simulink model "Arizona_base_GOAT_TjeerdRC"  (R2022a)
settings: Solver=FixedStepDiscrete  StartTime=0.0  StopTime=inf  FixedStep=Ts  RelTol=1e-3  EnableMultiTasking=on
undefined symbols (not defined in the file): DiscIntNeverNeededParam, Ended, IO307, N_Init, Nref, phd, phi_Init, Single, x_Init, y_Init
libraries: speedgoatlib_fpga_dio x30, speedgoatlib_fpga_quadrature x19, simulink x10, speedgoatlib_IO141 x9, xpcobsoletelib x7, cstblocks x5, speedgoatlib_fpga x3
(part 2 of 3)

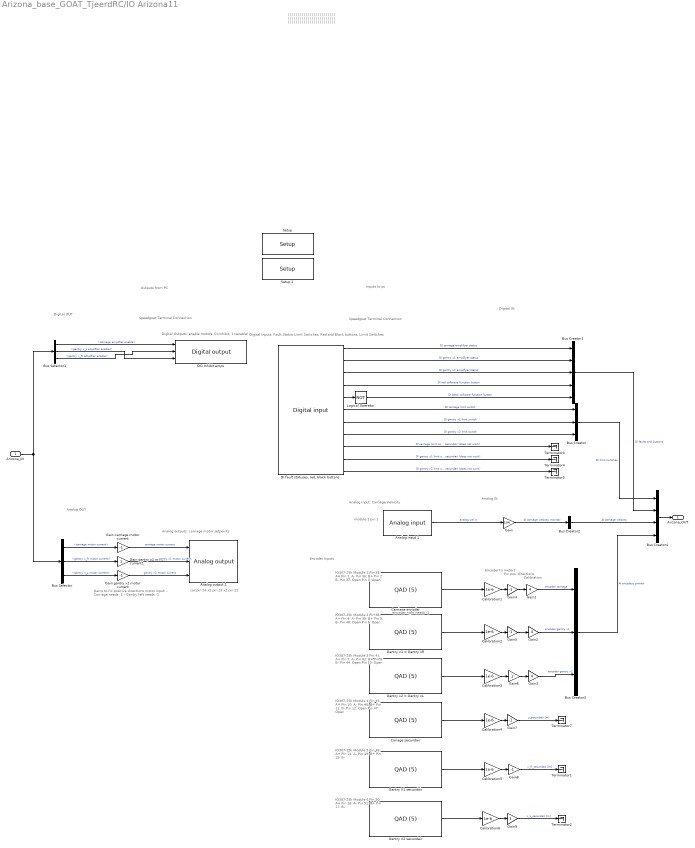
== system Arizona_base_GOAT_TjeerdRC/IO Arizona11 ==
  note: Fix pos.
      | directions
  note: Gains to fix positive directions motor input:
      | - Carriage needs -1
      | - Gantry left needs -1
  note: Inputs to pc
  note: Analog IN
  note: Digital IN
  note: Speedgoat Terminal Connection
  note: Outputs from PC
  note: Speedgoat Terminal Connection
  note: Digital Inputs: Fault Status Limit Switches, Red and Black buttons, Limit Switches
  note: Analog input: Carriage Velocity
  note: module 1
      | pin 1
  note: Digital OUT
  note: Analog OUT
  note: Analog outputs: carriage motor setpoints
  note: car pin 24
      | x1 pin 23
      | x2 pin 22
  note: |
      | |
      | |
      | |
      | |
      | |
      | |
      | |
      | |
      | |
      | |
      | |
      | |
      | |
      | |
      | |
      | |
      | |
      | |
      | |
      | |
      | |
      | |
      | |
      | |
      | |
      | |
      | |
      | |
      | |
      | |
      | |
      | |
      | |
      | |
      | |
      | |
      | |
      | |
      | |
      | |
      | |
      | |
      | |
      | |
      | |
      | |
      | |
      | |
      | |
      | |
      | |
      | |
      | |
      | |
      | |
      | |
      | |
      | |
      | |
      | |
      | |
      | |
      | |
      | |
      | |
      | |
      | |
      | |
      | |
      | |
      | |
  note: Digital Outputs: enable motors: 0=inhibit; 1=enable!
  note: Encoder
      | to meters
  note: Encoder Inputs
  note: encoder right needs -1
  note: IO307-25k
      | Module 4
      | Pin 45: A+
      | Pin 10: A-
      | Pin 46: B+
      | Pin 11: B-
      | Pin 12: Open
      | Pin 47: Open
  note: IO307-25k
      | Module 6
      | Pin 50: A+
      | Pin 16: A-
      | Pin 51: B+
      | Pin 17: B-
  note: IO307-25k
      | Module 3
      | Pin 41: A+
      | Pin 7: A-
      | Pin 42: B+
      | Pin 8: B-
      | Pin 44: Open
      | Pin 10: Open
  note: IO307-25k
      | Module 2
      | Pin 38: A+
      | Pin 4: A-
      | Pin 39: B+
      | Pin 5: B-
      | Pin 40: Open
      | Pin 6: Open
  note: IO307-25k
      | Module 5
      | Pin 48: A+
      | Pin 14: A-
      | Pin 49: B+
      | Pin 15: B-
  note: IO307-25k
      | Module 1
      | Pin 35: A+
      | Pin 1: A-
      | Pin 36: B+
      | Pin 2: B-
      | Pin 37: Open
      | Pin 3: Open
  note: Calibration
  Arizona_IN : Inport
  Analog input 1 : speedgoatlib_IO141/Analog input   parModuleId=1  parSampleTime=Ts  parPciSlot=-1  parAdcChannels=4  parAdcNumActiveChannels=[1 0]  parAdcVoltageRange=[5 5 5 5 5 5 5 5 5 5 5 5 5 5 5 5]  parAdcCoupling=[2 1]  parAdcContSampling=0  parAdcDmaEnable=0  parAdcActiveDmaDevices=[1 1 1 1]  parAdcFrameSize=100
      settings: SourceProductName=Simulink Real-Time: Speedgoat I/O Blockset
  Analog output 2 : speedgoatlib_IO141/Analog output   parModuleId=1  parSampleTime=Ts  parPciSlot=-1  parDacChannels=[1 2 3]  parDacVoltageRange=[5 5 5 7]  parDacOverRange=[0 0 0 0]  parDacInitValues=[0 0 0]  parDacReset=[1 1 1]  parDacSyncOut=1  parDacDmaEnable=0  parDacActiveDmaDevices=[1 1 1 1]  parDacDmaLatency=1  parDacFrameSize=100
      settings: SourceProductName=Simulink Real-Time: Speedgoat I/O Blockset
  Bus Creator : BusCreator  Inputs=3
  Bus Creator1 : BusCreator  Inputs=5
  Bus Creator2 : BusCreator  Inputs=1
  Bus Creator3 : BusCreator  Inputs=3
  Bus Creator4 : BusCreator  Inputs=4
  Bus Selector : BusSelector  OutputSignals=carriage motor current,gantry x_R motor current,gantry x_L motor current
  Bus Selector1 : BusSelector  OutputSignals=carriage amplifier enable,gantry x_L amplifier enable,gantry x_R amplifier enable
  Calibration{1..6} (6 alike) : Gain  Gain=1e-6
  Cariage secundair : speedgoatlib_fpga_quadrature/QAD (5)  id=1  chan=[4]  sampleTime=0.001  enableDma=on  board=Please select...  pciSlot=-1  numOfSlots=[1]  sensorType=Capture A + B Signal  interpolatePosition=off  swapAB=off  indexControlMode=Ignore Index  latchMode=Disabled  gateIndex=No Gating  speedFilterWidth=4  showInputSpeedFilterWidth=off  glitchFilterSeconds=106.7e-9  glitchFilterSecondsEff=108.5e-9  showInputClearPosition=off  showInputClearIndexFound=off  showOutputPosition=off  showOutputTurn=on  showOutputSpeed=off  showOutputIndexFound=off  showOutputLastPulse=off
      settings: SourceProductName=Simulink Real-Time: Speedgoat I/O Blockset
  Carriage encoder : speedgoatlib_fpga_quadrature/QAD (5)  id=1  chan=[1]  sampleTime=0.001  enableDma=on  board=Please select...  pciSlot=-1  numOfSlots=[1]  sensorType=Capture A + B Signal  interpolatePosition=off  swapAB=off  indexControlMode=Ignore Index  latchMode=Disabled  gateIndex=No Gating  speedFilterWidth=4  showInputSpeedFilterWidth=off  glitchFilterSeconds=106.7e-9  glitchFilterSecondsEff=108.5e-9  showInputClearPosition=off  showInputClearIndexFound=off  showOutputPosition=off  showOutputTurn=on  showOutputSpeed=off  showOutputIndexFound=off  showOutputLastPulse=off
      settings: SourceProductName=Simulink Real-Time: Speedgoat I/O Blockset
  "DI fault statuses, red, black buttons" : speedgoatlib_fpga_dio/Digital input  id=1  chan=[33:37,41:46]  ts=Ts  pciSlot=-1  board=IO307-25k  vectorizeOutput=off
      settings: SourceProductName=Simulink Real-Time: Speedgoat I/O Blockset
  DO Inhibit amps : speedgoatlib_fpga_dio/Digital output  id=1  chan=[30,31,32]  init=[0]  reset=[0]  vectorizeInput=off  ts=Ts  pciSlot=-1  board=Please select...
      settings: SourceProductName=Simulink Real-Time: Speedgoat I/O Blockset
  Gain : Gain  Gain=134
  Gain carriage motor current : Gain  Gain=-1
  Gain gantry x2 motor current : Gain  Gain=-1
  Gain gantry x2 motor current1 : Gain
  Gain1 : Gain  Gain=4
  Gain2 : Gain  Gain=4
  Gain3 : Gain  Gain=4
  Gain{4..5,7..8} (4 alike) : Gain  Gain=-1
  Gain6 : Gain
  Gain9 : Gain
  Gantry X1 secundair : speedgoatlib_fpga_quadrature/QAD (5)  id=1  chan=[5]  sampleTime=0.001  enableDma=on  board=Please select...  pciSlot=-1  numOfSlots=[1]  sensorType=Capture A + B Signal  interpolatePosition=off  swapAB=off  indexControlMode=Ignore Index  latchMode=Disabled  gateIndex=No Gating  speedFilterWidth=4  showInputSpeedFilterWidth=off  glitchFilterSeconds=106.7e-9  glitchFilterSecondsEff=108.5e-9  showInputClearPosition=off  showInputClearIndexFound=off  showOutputPosition=off  showOutputTurn=on  showOutputSpeed=off  showOutputIndexFound=off  showOutputLastPulse=off
      settings: SourceProductName=Simulink Real-Time: Speedgoat I/O Blockset
  Gantry x1 = Gantry xR : speedgoatlib_fpga_quadrature/QAD (5)  id=1  chan=[2]  sampleTime=0.001  enableDma=on  board=Please select...  pciSlot=-1  numOfSlots=[1]  sensorType=Capture A + B Signal  interpolatePosition=off  swapAB=off  indexControlMode=Ignore Index  latchMode=Disabled  gateIndex=No Gating  speedFilterWidth=4  showInputSpeedFilterWidth=off  glitchFilterSeconds=106.7e-9  glitchFilterSecondsEff=108.5e-9  showInputClearPosition=off  showInputClearIndexFound=off  showOutputPosition=off  showOutputTurn=on  showOutputSpeed=off  showOutputIndexFound=off  showOutputLastPulse=off
      settings: SourceProductName=Simulink Real-Time: Speedgoat I/O Blockset
  Gantry x2 = Gantry xL : speedgoatlib_fpga_quadrature/QAD (5)  id=1  chan=[3]  sampleTime=0.001  enableDma=on  board=Please select...  pciSlot=-1  numOfSlots=[1]  sensorType=Capture A + B Signal  interpolatePosition=off  swapAB=off  indexControlMode=Ignore Index  latchMode=Disabled  gateIndex=No Gating  speedFilterWidth=4  showInputSpeedFilterWidth=off  glitchFilterSeconds=106.7e-9  glitchFilterSecondsEff=108.5e-9  showInputClearPosition=off  showInputClearIndexFound=off  showOutputPosition=off  showOutputTurn=on  showOutputSpeed=off  showOutputIndexFound=off  showOutputLastPulse=off
      settings: SourceProductName=Simulink Real-Time: Speedgoat I/O Blockset
  Gentry X2 secundair : speedgoatlib_fpga_quadrature/QAD (5)  id=1  chan=[6]  sampleTime=0.001  enableDma=on  board=Please select...  pciSlot=-1  numOfSlots=[1]  sensorType=Capture A + B Signal  interpolatePosition=off  swapAB=off  indexControlMode=Ignore Index  latchMode=Disabled  gateIndex=No Gating  speedFilterWidth=4  showInputSpeedFilterWidth=off  glitchFilterSeconds=106.7e-9  glitchFilterSecondsEff=108.5e-9  showInputClearPosition=off  showInputClearIndexFound=off  showOutputPosition=off  showOutputTurn=on  showOutputSpeed=off  showOutputIndexFound=off  showOutputLastPulse=off
      settings: SourceProductName=Simulink Real-Time: Speedgoat I/O Blockset
  Logical Operator : Logic  Operator=NOT  AllPortsSameDT=off  OutDataTypeStr=boolean
  Setup : speedgoatlib_fpga/Setup/Setup  board=IO307-25k  id=1  device_id=1  frontIO=None  rearIO=None  bitstreamFile=speedgoat_IO307_25k_CI_02479  rev=1.000000  timestamp_string=28/12/21 17:14:03  fpgaFreq=73.73 MHz  fpgaTick=13.56 ns  ProgSpiFlash=off  ProgBPIFlash=off  pciSlot=-1  PullRPort0=pull-up 3.3V  VioPort0=3.3V  PullRPort1=pull-up 3.3V  VioPort1=3.3V  PullRPort2=pull-up 3.3V  VioPort2=3.3V  PullRPort3=pull-up 3.3V  VioPort3=3.3V  PullRPort4=pull-up 3.3V  VioPort4=3.3V  PullRPort5=pull-up 3.3V  VioPort5=3.3V  PullRPort6=pull-up 3.3V  VioPort6=3.3V  PullRPort15=pull-up 3.3V  PullRPort31=pull-up 3.3V  PullRPort47=pull-up 3.3V  PullRPort63=pull-up 3.3V  diffLineTermination_1=on  diffLineTermination_2=on  diffLineTermination_3=on  diffLineTermination_4=on  diffLineTermination_5=on  diffLineTermination_6=on  diffLineTermination_7=on  diffLineTermination_8=on
      settings: SourceProductName=Simulink Real-Time: Speedgoat I/O Blockset
  Setup 2 : speedgoatlib_IO141/Setup   parPciSlot=-1  parModuleId=1  parInterModuleSync=Independent  parConvClockBaseRate=20MHz  parConvClock1Divider=20000  parConvClock2Divider=20000  parFrameTriggerEnable=off  parFrameTriggerDivider=10  parConvClock1BaseRate=1  parConvClock2BaseRate=1  parFrameTriggerClock=1  parAdcCoupling1=Single-Ended  parAdcChannels1=[1 2]  parAdcChannel11=off  parAdcChannel12=off  parAdcChannel13=off  parAdcChannel14=on  parAdcChannel15=off  parAdcChannel16=off  parAdcChannel17=off  parAdcChannel18=off  parAdcRangeAll1=+-10.24 V  parVoltageRangePerChannelEn1=off  parAdcRange11=+-0.64 V  parAdcRange12=+-0.64 V  parAdcRange13=+-0.64 V  parAdcRange14=+-0.64 V  parAdcRange15=+-0.64 V  parAdcRange16=+-0.64 V  parAdcRange17=+-0.64 V  parAdcRange18=+-0.64 V  parAdcCoupling2=Differential  parAdcChannels2=[9 10]  parAdcChannel21=off  parAdcChannel22=off  parAdcChannel23=off  parAdcChannel24=off  parAdcChannel25=off  parAdcChannel26=off  parAdcChannel27=off  parAdcChannel28=off  parAdcRangeAll2=+-10.24 V  parVoltageRangePerChannelEn2=off  parAdcRange21=+-0.64 V  parAdcRange22=+-0.64 V  parAdcRange23=+-0.64 V  parAdcRange24=+-0.64 V  parAdcRange25=+-0.64 V  parAdcRange26=+-0.64 V  parAdcRange27=+-0.64 V  parAdcRange28=+-0.64 V  parAdcChannels=4  parAdcNumActiveChannels=[1 0]  parAdcVoltageRange=[5 5 5 5 5 5 5 5 5 5 5 5 5 5 5 5]  parAdcCoupling=[2 1]  parAdcContSampling=off  parAdcAutoCorrection=on  parAdcDmaEnable=off  parAdcDmaClock=Clock 1  parAdcFrameSize_=100  parAdcSampleTime_=-1  parAdcActiveDmaDevices=[1 1 1 1]  parAdcFrameTriggerEnable=0  parAdcFrameSize=100  parAdcSampleTime=0.1  parDacChannels=[1 2]  parDacChannel1=on  parDacChannel2=on  parDacChannel3=on  parDacChannel4=off  parDacInitValues=0  parDacResets=1  parDacVoltageRange=[5 5 5 7]  parDacOverRange=[0 0 0 0]  parDacRange1=+-5 V  parDacInitValue1=0  parDacReset1=on  parDacRange2=+-5 V  parDacInitValue2=0  parDacReset2=on  parDacRange3=+-5 V  parDacInitValue3=0  parDacReset3=on  parDacRange4=+-10 V  parDacInitValue4=0  parDacReset4=on  parDacAutoCorrection=on  parDacSyncOut=on  parDacDmaEnable=off  parDacDmaLatency=As small as possible  parDacDmaClock=Clock 1  parDacFrameSize_=100  parDacSampleTime_=-1  parDacActiveDmaDevices=[1 1 1 1]  parDacFrameTriggerEnable=0  parDacFrameSize=100  parDacSampleTime=0.1  parDiChannels=[1 2 3 4 5]  parDoChannels=[6 7 8]  parDioChannel1=In  parDioChannel2=In  parDioChannel3=In  parDioChannel4=In  parDioChannel5=In  parDioChannel6=Out  parDioChannel7=Out  parDioChannel8=Out  parDoInitValues=[0 0 0]  parDoReset=[1 1 1]  parDoInitValue1=0  parDoReset1=on  parDoInitValue2=0  parDoReset2=on  parDoInitValue3=0  parDoReset3=on  parDoInitValue4=0  parDoReset4=on  parDoInitValue5=0  parDoReset5=on  parDoInitValue6=0  parDoReset6=on  parDoInitValue7=0  parDoReset7=on  parDoInitValue8=0  parDoReset8=on  parDiDebounceEnable=off  parDiDebounceTime=0  parDiDebounceValue=0  parDioPullRefFront=Pull-up 3.3 V  parDioPullRefRear=Floating
      settings: SourceProductName=Simulink Real-Time: Speedgoat I/O Blockset
  Terminator{1..5,7} (6 alike) : Terminator
  Arizona_OUT : Outport
  wires:
  "DI fault statuses, red, black buttons"/8 -> Bus Creator/3  "DI gantry x2 limit switch"
  Bus Creator3/1 -> Bus Creator4/4  "AI encoders primair"
  Bus Creator2/1 -> Bus Creator4/3  "AI carriage velocity"
  Bus Creator1/1 -> Bus Creator4/2  "DI faults and buttons"
  Bus Creator/1 -> Bus Creator4/1  "DI limit switches"
  Gain carriage motor current/1 -> Analog output 2/1  "carriage motor current"
  Bus Selector/3 -> Gain gantry x2 motor current/1  "<gantry x_L motor current>"
  "DI fault statuses, red, black buttons"/5 -> Logical Operator/1
  Logical Operator/1 -> Bus Creator1/5  "DI black sofware function button"
  "DI fault statuses, red, black buttons"/2 -> Bus Creator1/2  "DI gantry x1 amplifyer status"
  "DI fault statuses, red, black buttons"/3 -> Bus Creator1/3  "DI gantry x2 amplifyer status"
  Bus Selector/2 -> Gain gantry x2 motor current1/1  "<gantry x_R motor current>"
  "DI fault statuses, red, black buttons"/4 -> Bus Creator1/4  "DI red software function button"
  "DI fault statuses, red, black buttons"/7 -> Bus Creator/2  "DI gantry x1 limit switch"
  "DI fault statuses, red, black buttons"/1 -> Bus Creator1/1  "DI carriage amplifyer status"
  "DI fault statuses, red, black buttons"/6 -> Bus Creator/1  "DI carriage limit switch"
  Bus Selector/1 -> Gain carriage motor current/1  "<carriage motor current>"
  Gain gantry x2 motor current/1 -> Analog output 2/3  "gantry x2 motor current"
  Gain/1 -> Bus Creator2/1  "AI carriage velocity monitor"
  Bus Creator4/1 -> Arizona_OUT/1
  Gain gantry x2 motor current1/1 -> Analog output 2/2  "gantry x1 motor current"
  Analog input 1/1 -> Gain/1  "analog vel in"
  Bus Selector1/3 -> DO Inhibit amps/2  "<gantry x_R amplifier enable>"
  Arizona_IN/1 -> Bus Selector1/1, Bus Selector/1
  Bus Selector1/1 -> DO Inhibit amps/1  "<carriage amplifier enable>"
  Calibration2/1 -> Gain5/1
  Calibration3/1 -> Gain6/1
  Calibration1/1 -> Gain4/1
  Calibration4/1 -> Gain7/1
  Calibration5/1 -> Gain8/1
  Calibration6/1 -> Gain9/1
  "DI fault statuses, red, black buttons"/9 -> Terminator3/1  "DI carriage limit switch secundair (does not work)"
  "DI fault statuses, red, black buttons"/10 -> Terminator4/1  "DI gantry x1 limit switch secundair (does not work)"
  "DI fault statuses, red, black buttons"/11 -> Terminator5/1  "DI gantry x2 limit switch secundair (does not work)"
  Bus Selector1/2 -> DO Inhibit amps/3  "<gantry x_L amplifier enable>"
  Gain2/1 -> Bus Creator3/2  "encoder gantry x1"
  Gain3/1 -> Bus Creator3/3  "encoder gantry x2"
  Gain8/1 -> Terminator1/1  "x_R_secundair [m]"
  Gain9/1 -> Terminator2/1  "x_L_secundair [m]"
  Gain1/1 -> Bus Creator3/1  "encoder carriage"
  Gain7/1 -> Terminator7/1  "y_secundair [m]"
  Carriage encoder/1 -> Calibration1/1
  Gantry x1 = Gantry xR/1 -> Calibration2/1
  Gantry x2 = Gantry xL/1 -> Calibration3/1
  Cariage secundair/1 -> Calibration4/1
  Gantry X1 secundair/1 -> Calibration5/1
  Gentry X2 secundair/1 -> Calibration6/1
  Gain4/1 -> Gain1/1
  Gain5/1 -> Gain2/1
  Gain6/1 -> Gain3/1

== system Arizona_base_GOAT_TjeerdRC/Penholder mechanism1 ==
  note: -1= naar beneden
      | 1= omhoog
      | 0=uit
  note: -1=CCW
      | 1= CW
      | 0=uit
  note: LimitSwitch_z_up DI PF50 PIN 6 #CON-0 6229
  note: Limitswitch_z_down DI PFI14 PIN 1 #CON-0 6229
  note: LimitSwitch_Theta DI PFI9 PIN 3 #CON-0 6229
  Change color : Inport
  homingDone : Inport  Port=2
  Change color Chart : Stateflow chart  TreatAsAtomicUnit=on
  Data Type Conversion1 : DataTypeConversion  SaturateOnIntegerOverflow=off  RndMeth=Floor
  Data Type Conversion2 : DataTypeConversion  SaturateOnIntegerOverflow=off  RndMeth=Floor
  Data Type Conversion3 : DataTypeConversion  SaturateOnIntegerOverflow=off  RndMeth=Floor
  Gain on phi2 : Gain  Gain=0.07
  Gain on phi3 : Gain
  Motor Theta : Subsystem
  Motor Z : Subsystem
  "PCI 6229 PFI DI " : xpcobsoletelib/Obsolete  Commented=on
      settings: SourceProductBaseCode=XP
  PCI 6229 PFI DI 1 : xpcobsoletelib/Obsolete  Commented=on
      settings: SourceProductBaseCode=XP
  PCI 6229 PFI DI 2 : xpcobsoletelib/Obsolete  Commented=on
      settings: SourceProductBaseCode=XP
  log_jogspeed : Gain
  Penholder_active : Outport
  wires:
  ? -> Data Type Conversion1/1
  ? -> Data Type Conversion2/1
  Gain on phi2/1 -> Motor Theta/1(v_theta in mm/s)
  Gain on phi3/1 -> Motor Z/1(v_Z in mm/s)
  ? -> Data Type Conversion3/1
  Data Type Conversion3/1 -> Change color Chart/4(limitSwitch_Theta)
  Change color/1 -> Change color Chart/1(change_color)
  Change color Chart/1(jogspeed_Z) -> Gain on phi3/1
  Change color Chart/2(jogspeed_Theta) -> log_jogspeed/1
  Data Type Conversion2/1 -> Change color Chart/2(limitSwitch_z_up)
  Data Type Conversion1/1 -> Change color Chart/3(limitSwitch_z_down)
  Change color Chart/3(active) -> Penholder_active/1
  log_jogspeed/1 -> Gain on phi2/1  "jogSpeed"
  homingDone/1 -> Change color Chart/5(homingDone)

== system Arizona_base_GOAT_TjeerdRC/Repetitive Controller ==
  Learning Gain : Inport
  y : Inport  Port=2
  r : Inport  Port=3
  e : Inport  Port=4
  Enable : EnablePort
  Lc : cstblocks/LTI System  sys=Lc  IC=[]
  Product : Product
  Qc : cstblocks/LTI System  sys=Qc  IC=[]
  Sum : Sum  Inputs=|++
  z^(N-phd-p_Q) : Delay  DelayLength=Nlength-phd-p_Q
  z^-phd : Delay  DelayLength=phd
  Out1 : Outport
  wires:
  Sum/1 -> z^(N-phd-p_Q)/1
  e/1 -> Sum/1
  z^(N-phd-p_Q)/1 -> Qc/1
  Qc/1 -> z^-phd/1, Lc/1
  z^-phd/1 -> Sum/2
  Lc/1 -> Product/2
  Product/1 -> Out1/1
  Learning Gain/1 -> Product/1

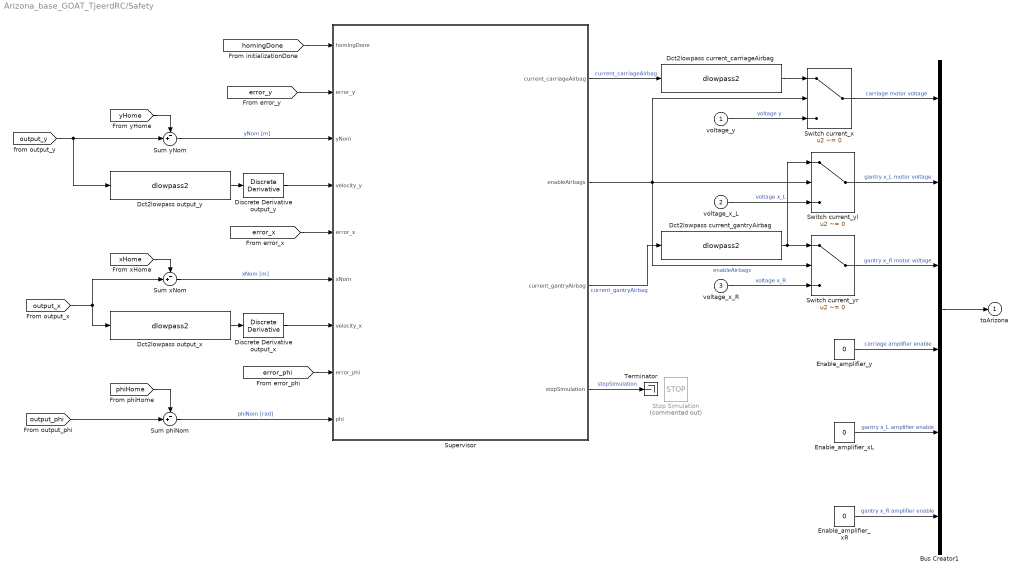
== system Arizona_base_GOAT_TjeerdRC/Safety ==
  voltage_y : Inport
  voltage_x_L : Inport  Port=2
  voltage_x_R : Inport  Port=3
  Bus Creator1 : BusCreator  Inputs=carriage motor voltage,gantry x_L motor voltage,gantry x_R motor voltage,carriage amplifier enable,gantry x_L amplifier enable,gantry x_R amplifier enable
  Dct2lowpass current_carriageAirbag : S-Function  FunctionName=dlowpass2  Parameters=f_den, b_den, 0.001  SFunctionDeploymentMode=off  EnableBusSupport=off  mask(dctools){f_den=5, b_den=2}
      mask prompts: f_den "Pole [Hz]"; b_den "Damping pole [-]"
      mask help: This block implements a discrete time 2nd order lowpass filter.
      mask Display: disp('DCT 2nd order lowpass')
  Dct2lowpass current_gantryAirbag : S-Function  FunctionName=dlowpass2  Parameters=f_den, b_den, 0.001  SFunctionDeploymentMode=off  EnableBusSupport=off  mask(dctools){f_den=5, b_den=2}
      mask prompts: f_den "Pole [Hz]"; b_den "Damping pole [-]"
      mask help: This block implements a discrete time 2nd order lowpass filter.
      mask Display: disp('DCT 2nd order lowpass')
  Dct2lowpass output_x : S-Function  FunctionName=dlowpass2  Parameters=f_den, b_den, 0.001  SFunctionDeploymentMode=off  EnableBusSupport=off  mask(dctools){f_den=10, b_den=2}
      mask prompts: f_den "Pole [Hz]"; b_den "Damping pole [-]"
      mask help: This block implements a discrete time 2nd order lowpass filter.
      mask Display: disp('DCT 2nd order lowpass')
  Dct2lowpass output_y : S-Function  FunctionName=dlowpass2  Parameters=f_den, b_den, 0.001  SFunctionDeploymentMode=off  EnableBusSupport=off  mask(dctools){f_den=10, b_den=2}
      mask prompts: f_den "Pole [Hz]"; b_den "Damping pole [-]"
      mask help: This block implements a discrete time 2nd order lowpass filter.
      mask Display: disp('DCT 2nd order lowpass')
  Discrete Derivative output_x : simulink/Discrete/Discrete Derivative  gainval=1.0  ICPrevScaledInput=0.0  OutMin=[]  OutMax=[]  OutDataType=fixdt(1, 16)  OutScaling=2^-10  DoSatur=off
  Discrete Derivative output_y : simulink/Discrete/Discrete Derivative  gainval=1.0  ICPrevScaledInput=0.0  OutMin=[]  OutMax=[]  OutDataType=fixdt(1, 16)  OutScaling=2^-10  DoSatur=off
  Enable_amplifier_xL : Constant  Value=0
  Enable_amplifier_xR : Constant  Value=0
  Enable_amplifier_y : Constant  Value=0
  Stop Simulation : Stop  Commented=on
  Sum phiNom : Sum  Inputs=-+|
  Sum xNom : Sum  Inputs=-+|
  Sum yNom : Sum  Inputs=-+|
  Supervisor : Stateflow chart  TreatAsAtomicUnit=on
  Switch current_x : Switch  Criteria=u2 ~= 0  SaturateOnIntegerOverflow=off  InputSameDT=off
  Switch current_yl : Switch  Criteria=u2 ~= 0  SaturateOnIntegerOverflow=off  InputSameDT=off
  Switch current_yr : Switch  Criteria=u2 ~= 0  SaturateOnIntegerOverflow=off  InputSameDT=off
  Terminator : Terminator
  toArizona : Outport
  wires:
  [phiHome] -> Sum phiNom/1
  Sum phiNom/1 -> Supervisor/9(phi)  "phiNom [rad]"
  voltage_x_L/1 -> Switch current_yl/3  "voltage x_L"
  voltage_x_R/1 -> Switch current_yr/3  "voltage x_R"
  Dct2lowpass current_carriageAirbag/1 -> Switch current_x/1
  Dct2lowpass current_gantryAirbag/1 -> Switch current_yl/1, Switch current_yr/1
  Supervisor/3(current_gantryAirbag) -> Dct2lowpass current_gantryAirbag/1  "current_gantryAirbag"
  Discrete Derivative output_x/1 -> Supervisor/7(velocity_x)
  [xHome] -> Sum xNom/1
  Dct2lowpass output_x/1 -> Discrete Derivative output_x/1
  Sum xNom/1 -> Supervisor/6(xNom)  "xNom [m]"
  [output_x] -> Sum xNom/2, Dct2lowpass output_x/1
  [error_phi] -> Supervisor/8(error_phi)
  [error_x] -> Supervisor/5(error_x)
  Supervisor/2(enableAirbags) -> Switch current_yr/2, Switch current_yl/2, Switch current_x/2  "enableAirbags"
  Supervisor/1(current_carriageAirbag) -> Dct2lowpass current_carriageAirbag/1  "current_carriageAirbag"
  [error_y] -> Supervisor/2(error_y)
  Switch current_x/1 -> Bus Creator1/1  "carriage motor voltage"
  [homingDone] -> Supervisor/1(homingDone)
  [yHome] -> Sum yNom/1
  voltage_y/1 -> Switch current_x/3  "voltage y"
  Discrete Derivative output_y/1 -> Supervisor/4(velocity_y)
  Dct2lowpass output_y/1 -> Discrete Derivative output_y/1
  Sum yNom/1 -> Supervisor/3(yNom)  "yNom [m]"
  [output_y] -> Dct2lowpass output_y/1, Sum yNom/2
  Bus Creator1/1 -> toArizona/1
  Enable_amplifier_xL/1 -> Bus Creator1/5  "gantry x_L amplifier enable"
  Enable_amplifier_xR/1 -> Bus Creator1/6  "gantry x_R amplifier enable"
  Switch current_yl/1 -> Bus Creator1/2  "gantry x_L motor voltage"
  Enable_amplifier_y/1 -> Bus Creator1/4  "carriage amplifier enable"
  Switch current_yr/1 -> Bus Creator1/3  "gantry x_R motor voltage"
  [output_phi] -> Sum phiNom/2
  Supervisor/4(stopSimulation) -> Terminator/1  "stopSimulation"

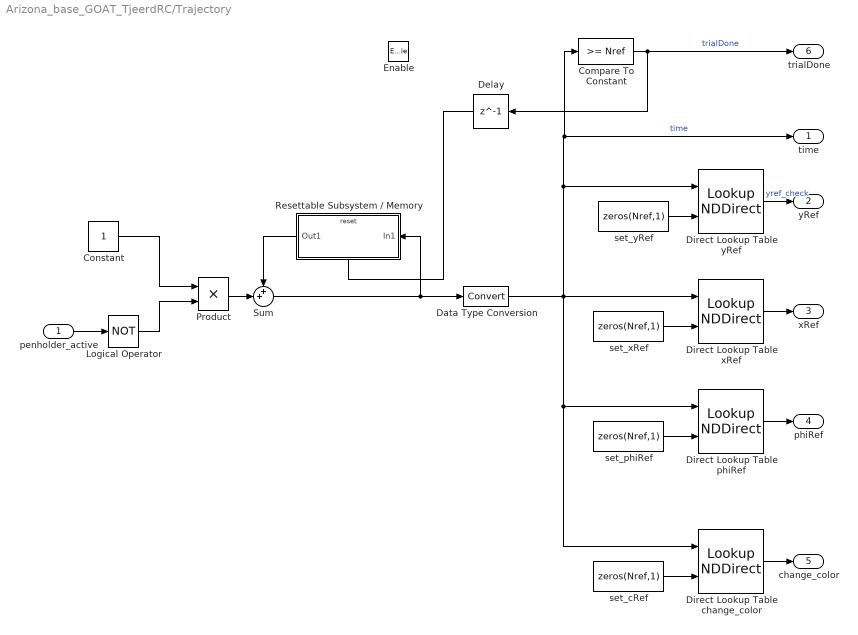
== system Arizona_base_GOAT_TjeerdRC/Trajectory ==
  penholder_active : Inport
  Enable : EnablePort  StatesWhenEnabling=reset
  Compare To Constant : simulink/Logic and Bit Operations/Compare To Constant  relop=>=  const=Nref  OutDataTypeStr=boolean
  Constant : Constant
  Data Type Conversion : DataTypeConversion  SaturateOnIntegerOverflow=off  RndMeth=Floor
  Delay : Delay  DelayLength=1  InitialCondition=0
  Direct Lookup Table change_color : LookupNDDirect  NumberOfTableDimensions=1  TableIsInput=on  Table=[4 5 ;16 19 ]
  Direct Lookup Table phiRef : LookupNDDirect  NumberOfTableDimensions=1  TableIsInput=on  Table=[4 5 ;16 19 ]
  Direct Lookup Table xRef : LookupNDDirect  NumberOfTableDimensions=1  TableIsInput=on  Table=[4 5 ;16 19 ]
  Direct Lookup Table yRef : LookupNDDirect  NumberOfTableDimensions=1  TableIsInput=on  Table=[4 5 ;16 19 ]
  Logical Operator : Logic  Operator=NOT  AllPortsSameDT=off  OutDataTypeStr=boolean
  Product : Product
  Resettable Subsystem / Memory : Subsystem  TreatAsAtomicUnit=on
  Sum : Sum  Inputs=++|
  set_cRef : Constant  Value=zeros(Nref,1)
  set_phiRef : Constant  Value=zeros(Nref,1)
  set_xRef : Constant  Value=zeros(Nref,1)
  set_yRef : Constant  Value=zeros(Nref,1)
  time : Outport
  yRef : Outport  Port=2
  xRef : Outport  Port=3
  phiRef : Outport  Port=4
  change_color : Outport  Port=5
  trialDone : Outport  Port=6
  wires:
  Direct Lookup Table phiRef/1 -> phiRef/1
  Direct Lookup Table yRef/1 -> yRef/1  "yref_check"
  Direct Lookup Table xRef/1 -> xRef/1
  set_yRef/1 -> Direct Lookup Table yRef/2
  set_xRef/1 -> Direct Lookup Table xRef/2
  Data Type Conversion/1 -> Compare To Constant/1, time/1, Direct Lookup Table yRef/1, Direct Lookup Table xRef/1, Direct Lookup Table change_color/1, Direct Lookup Table phiRef/1  "time"
  set_phiRef/1 -> Direct Lookup Table phiRef/2
  Constant/1 -> Product/1
  Sum/1 -> Resettable Subsystem / Memory/1(In1), Data Type Conversion/1
  penholder_active/1 -> Logical Operator/1
  Logical Operator/1 -> Product/2
  Direct Lookup Table change_color/1 -> change_color/1
  set_cRef/1 -> Direct Lookup Table change_color/2
  Compare To Constant/1 -> Delay/1, trialDone/1  "trialDone"
  Product/1 -> Sum/2
  Resettable Subsystem / Memory/1(Out1) -> Sum/1
  Delay/1 -> Resettable Subsystem / Memory/Reset

== system Arizona_base_GOAT_TjeerdRC/Homing/Enabled subsystem ==
  encoderSignals : Inport
  penholder_active : Inport  Port=2
  Enable : EnablePort  StatesWhenEnabling=reset
  Add phiHome : Sum  Inputs=|++
  Add xHome : Sum  Inputs=|++
  Add yHome : Sum  Inputs=|++
  Initialization : Subsystem
  Reset : Subsystem
  yHome : Outport
  xHome : Outport  Port=2
  phiHome : Outport  Port=3
  homingDone : Outport  Port=4  InitialOutput=0
  change_color : Outport  Port=5
  wires:
  encoderSignals/1 -> Reset/1(encoderSignals)
  Reset/1(yReset) -> Add yHome/1  "yReset"
  Reset/2(xReset) -> Add xHome/1  "xReset"
  Reset/3(phiReset) -> Add phiHome/1  "phiReset"
  Initialization/4(initializationDone) -> homingDone/1
  Add xHome/1 -> xHome/1
  Add yHome/1 -> yHome/1
  Add phiHome/1 -> phiHome/1
  penholder_active/1 -> Reset/2(penholder_active)
  Reset/5(change_color) -> change_color/1
  Initialization/3(phiInit) -> Add phiHome/2  "phiInit"
  Initialization/1(yInit) -> Add yHome/2  "yInit"
  Initialization/2(xInit) -> Add xHome/2  "xInit"
  Reset/4(resetDone) -> Initialization/1(resetDone)  "resetDone"

== system Arizona_base_GOAT_TjeerdRC/Homing/Memory block for homing during trials ==
  yHome : Inport
  xHome : Inport  Port=2
  phiHome : Inport  Port=3
  homeTrigger : Inport  Port=4
  Memory_phi : Subsystem
  Memory_x : Subsystem
  Memory_y : Subsystem
  yHome_memory : Outport
  xHome_memory : Outport  Port=2
  phiHome_memory : Outport  Port=3
  wires:
  yHome/1 -> Memory_y/2(yHome)
  xHome/1 -> Memory_x/2(xHome)
  phiHome/1 -> Memory_phi/2(phiHome)
  homeTrigger/1 -> Memory_phi/1(homeTrigger), Memory_x/1(homeTrigger), Memory_y/1(homeTrigger)
  Memory_y/1(Out1) -> yHome_memory/1
  Memory_x/1(1) -> xHome_memory/1
  Memory_phi/1(1) -> phiHome_memory/1

== system Arizona_base_GOAT_TjeerdRC/Homing old/Enabled subsystem ==
  encoderSignals : Inport
  penholder_active : Inport  Port=2
  Enable : EnablePort  StatesWhenEnabling=reset
  Add phiHome : Sum  Inputs=|++
  Add xHome : Sum  Inputs=|++
  Add yHome : Sum  Inputs=|++
  Initialization : Subsystem  TreatAsAtomicUnit=on
  Reset : Subsystem
  yHome : Outport
  xHome : Outport  Port=2
  phiHome : Outport  Port=3
  homingDone : Outport  Port=4  InitialOutput=0
  change_color : Outport  Port=5
  wires:
  encoderSignals/1 -> Reset/1(encoderSignals)
  Reset/4(resetDone) -> Initialization/Enable
  Reset/1(yReset) -> Add yHome/1  "yReset"
  Reset/2(xReset) -> Add xHome/1  "xReset"
  Reset/3(phiReset) -> Add phiHome/1  "phiReset"
  Initialization/4(initializationDone) -> homingDone/1
  Add xHome/1 -> xHome/1
  Add yHome/1 -> yHome/1
  Add phiHome/1 -> phiHome/1
  penholder_active/1 -> Reset/2(penholder_active)
  Reset/5(change_color) -> change_color/1
  Initialization/3(phiInit) -> Add phiHome/2  "phiInit"
  Initialization/1(yInit) -> Add yHome/2  "yInit"
  Initialization/2(xInit) -> Add xHome/2  "xInit"

== system Arizona_base_GOAT_TjeerdRC/Homing old/Memory ==
  homeTrigger : Inport
  yHome : Inport  Port=2
  Delay : Delay  DelayLength=1
  Memory : Memory
  Sum : Sum  Inputs=|++
  Switch : Switch  Criteria=u2 > Threshold  Threshold=1  SaturateOnIntegerOverflow=off  InputSameDT=off
  Switch1 : Switch  Criteria=u2 > Threshold  SaturateOnIntegerOverflow=off  InputSameDT=off
  Out1 : Outport
  wires:
  Switch/1 -> Memory/1
  Memory/1 -> Switch/3, Switch1/3, Sum/2
  homeTrigger/1 -> Delay/1, Switch1/2
  yHome/1 -> Sum/1
  Sum/1 -> Switch1/1
  Switch1/1 -> Switch/1, Out1/1
  Delay/1 -> Switch/2

== system Arizona_base_GOAT_TjeerdRC/Penholder mechanism1/Motor Theta ==
  note: enable DO PFI4 PIN 41 #CON-0 6229
  note: direction DO PFI3 PIN 42 #CON-0 6229
  v_theta in mm/s : Inport
  Abs : Abs  SaturateOnIntegerOverflow=off
  Compare To Zero : simulink/Logic and Bit Operations/Compare To Zero  relop=>  OutDataTypeStr=boolean
  Data Type Conversion : DataTypeConversion  SaturateOnIntegerOverflow=off  RndMeth=Floor
  "PCI 6229 PFI DO " : xpcobsoletelib/Obsolete  Commented=on
      settings: SourceProductBaseCode=XP
  PCI 6229 PWM Generate Chan 0 : xpcobsoletelib/Obsolete  Commented=on
      settings: SourceProductBaseCode=XP
  PWMcreator5 : Subsystem
  wires:
  PWMcreator5/1(HighSamples) -> ?
  PWMcreator5/2(LowSamples) -> ?
  Compare To Zero/1 -> Data Type Conversion/1
  PWMcreator5/3(DirectionBit) -> ?
  Data Type Conversion/1 -> ?
  Abs/1 -> Compare To Zero/1
  v_theta in mm/s/1 -> Abs/1, PWMcreator5/1(velocity [mm / s])

== system Arizona_base_GOAT_TjeerdRC/Penholder mechanism1/Motor Z ==
  note: enable DO PFI11 PIN 46 #CON-0 6229
  note: direction DO PFI10 PIN 45 #CON-0 6229
  v_Z in mm/s : Inport
  Abs1 : Abs  SaturateOnIntegerOverflow=off
  Compare To Zero1 : simulink/Logic and Bit Operations/Compare To Zero  relop=>  OutDataTypeStr=boolean
  Data Type Conversion1 : DataTypeConversion  SaturateOnIntegerOverflow=off  RndMeth=Floor
  PCI 6229 PFI DO 1 : xpcobsoletelib/Obsolete  Commented=on
      settings: SourceProductBaseCode=XP
  PCI 6229 PWM Generate Chan 1 : xpcobsoletelib/Obsolete  Commented=on
      settings: SourceProductBaseCode=XP
  PWMcreator1 : Subsystem
  wires:
  PWMcreator1/1(HighSamples) -> ?
  PWMcreator1/2(LowSamples) -> ?
  Compare To Zero1/1 -> Data Type Conversion1/1
  PWMcreator1/3(DirectionBit) -> ?
  v_Z in mm/s/1 -> Abs1/1, PWMcreator1/1(velocity [mm / s])
  Data Type Conversion1/1 -> ?
  Abs1/1 -> Compare To Zero1/1

== system Arizona_base_GOAT_TjeerdRC/Trajectory/Resettable Subsystem // Memory ==
  In1 : Inport
  Reset : ResetPort  DisableCoverage=on
  Memory : Memory
  Out1 : Outport
  wires:
  In1/1 -> Memory/1
  Memory/1 -> Out1/1

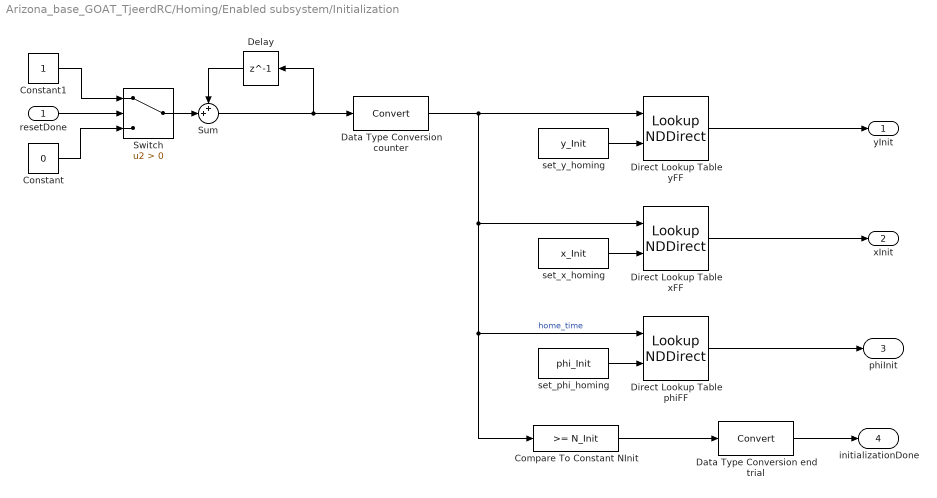
== system Arizona_base_GOAT_TjeerdRC/Homing/Enabled subsystem/Initialization ==
  resetDone : Inport
  Compare To Constant NInit : simulink/Logic and Bit Operations/Compare To Constant  relop=>=  const=N_Init  OutDataTypeStr=boolean
  Constant : Constant  Value=0
  Constant1 : Constant
  Data Type Conversion counter : DataTypeConversion  SaturateOnIntegerOverflow=off  RndMeth=Floor
  Data Type Conversion end trial : DataTypeConversion  SaturateOnIntegerOverflow=off  RndMeth=Floor
  Delay : Delay  DelayLength=1
  Direct Lookup Table phiFF : LookupNDDirect  NumberOfTableDimensions=1  TableIsInput=on  Table=[4 5 ;16 19 ]
  Direct Lookup Table xFF : LookupNDDirect  NumberOfTableDimensions=1  TableIsInput=on  Table=[4 5 ;16 19 ]
  Direct Lookup Table yFF : LookupNDDirect  NumberOfTableDimensions=1  TableIsInput=on  Table=[4 5 ;16 19 ]
  Sum : Sum  Inputs=++|
  Switch : Switch  Criteria=u2 > Threshold  SaturateOnIntegerOverflow=off  InputSameDT=off
  set_phi_homing : Constant  Value=phi_Init
  set_x_homing : Constant  Value=x_Init
  set_y_homing : Constant  Value=y_Init
  yInit : Outport
  xInit : Outport  Port=2
  phiInit : Outport  Port=3
  initializationDone : Outport  Port=4
  wires:
  Data Type Conversion counter/1 -> Direct Lookup Table xFF/1, Direct Lookup Table phiFF/1, Compare To Constant NInit/1, Direct Lookup Table yFF/1  "home_time"
  set_phi_homing/1 -> Direct Lookup Table phiFF/2
  Direct Lookup Table yFF/1 -> yInit/1
  set_x_homing/1 -> Direct Lookup Table xFF/2
  Direct Lookup Table xFF/1 -> xInit/1
  Compare To Constant NInit/1 -> Data Type Conversion end trial/1
  Data Type Conversion end trial/1 -> initializationDone/1
  Direct Lookup Table phiFF/1 -> phiInit/1
  set_y_homing/1 -> Direct Lookup Table yFF/2
  resetDone/1 -> Switch/2
  Constant/1 -> Switch/3
  Constant1/1 -> Switch/1
  Switch/1 -> Sum/2
  Sum/1 -> Data Type Conversion counter/1, Delay/1
  Delay/1 -> Sum/1

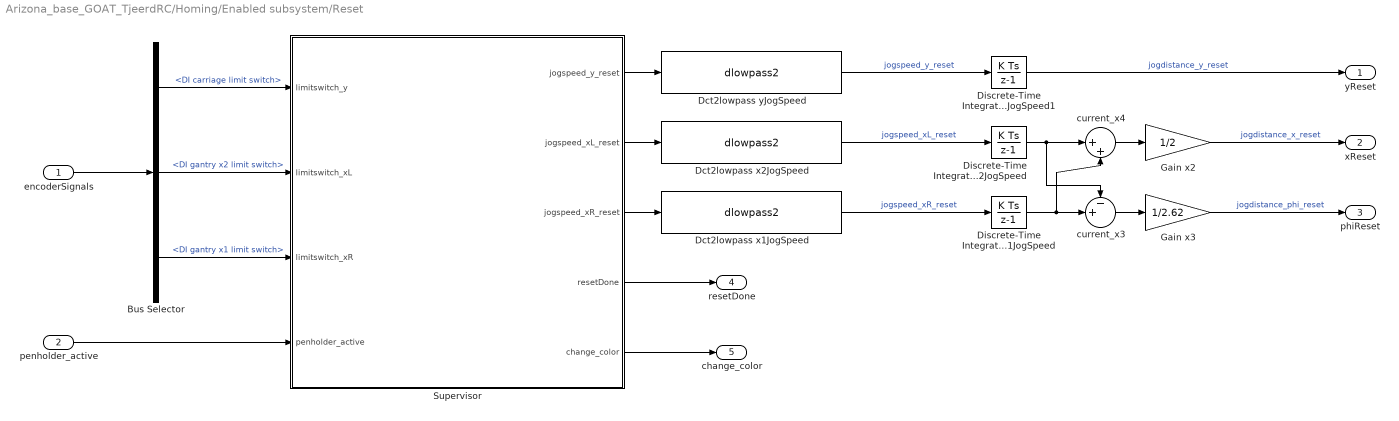
== system Arizona_base_GOAT_TjeerdRC/Homing/Enabled subsystem/Reset ==
  encoderSignals : Inport
  penholder_active : Inport  Port=2
  Bus Selector : BusSelector  OutputSignals=DI limit switches.DI carriage limit switch,DI limit switches.DI gantry x2 limit switch,DI limit switches.DI gantry x1 limit switch
  Dct2lowpass x1JogSpeed : S-Function  FunctionName=dlowpass2  Parameters=f_den, b_den, 0.001  SFunctionDeploymentMode=off  EnableBusSupport=off  mask(dctools){f_den=20, b_den=2}
      mask prompts: f_den "Pole [Hz]"; b_den "Damping pole [-]"
      mask help: This block implements a discrete time 2nd order lowpass filter.
      mask Display: disp('DCT 2nd order lowpass')
  Dct2lowpass x2JogSpeed : S-Function  FunctionName=dlowpass2  Parameters=f_den, b_den, 0.001  SFunctionDeploymentMode=off  EnableBusSupport=off  mask(dctools){f_den=20, b_den=2}
      mask prompts: f_den "Pole [Hz]"; b_den "Damping pole [-]"
      mask help: This block implements a discrete time 2nd order lowpass filter.
      mask Display: disp('DCT 2nd order lowpass')
  Dct2lowpass yJogSpeed : S-Function  FunctionName=dlowpass2  Parameters=f_den, b_den, 0.001  SFunctionDeploymentMode=off  EnableBusSupport=off  mask(dctools){f_den=10, b_den=1}
      mask prompts: f_den "Pole [Hz]"; b_den "Damping pole [-]"
      mask help: This block implements a discrete time 2nd order lowpass filter.
      mask Display: disp('DCT 2nd order lowpass')
  Discrete-Time Integrator x1JogSpeed : DiscreteIntegrator  SampleTime=-1  ICPrevOutput=DiscIntNeverNeededParam  ICPrevScaledInput=DiscIntNeverNeededParam
  Discrete-Time Integrator x2JogSpeed : DiscreteIntegrator  SampleTime=-1  ICPrevOutput=DiscIntNeverNeededParam  ICPrevScaledInput=DiscIntNeverNeededParam
  Discrete-Time Integrator x2JogSpeed1 : DiscreteIntegrator  SampleTime=-1  ICPrevOutput=DiscIntNeverNeededParam  ICPrevScaledInput=DiscIntNeverNeededParam
  Gain x2 : Gain  Gain=1/2  OutDataTypeStr=double
  Gain x3 : Gain  Gain=1/2.62  OutDataTypeStr=double
  Supervisor : Stateflow chart  TreatAsAtomicUnit=on
  current_x3 : Sum  Inputs=-+|
  current_x4 : Sum  Inputs=|++
  yReset : Outport
  xReset : Outport  Port=2
  phiReset : Outport  Port=3
  resetDone : Outport  Port=4
  change_color : Outport  Port=5
  wires:
  Bus Selector/3 -> Supervisor/3(limitswitch_xR)  "<DI gantry x1 limit switch>"
  Gain x2/1 -> xReset/1  "jogdistance_x_reset"
  encoderSignals/1 -> Bus Selector/1
  Supervisor/4(resetDone) -> resetDone/1
  Supervisor/2(jogspeed_xL_reset) -> Dct2lowpass x2JogSpeed/1
  Supervisor/3(jogspeed_xR_reset) -> Dct2lowpass x1JogSpeed/1
  Dct2lowpass x2JogSpeed/1 -> Discrete-Time Integrator x2JogSpeed/1  "jogspeed_xL_reset"
  Dct2lowpass x1JogSpeed/1 -> Discrete-Time Integrator x1JogSpeed/1  "jogspeed_xR_reset"
  Bus Selector/2 -> Supervisor/2(limitswitch_xL)  "<DI gantry x2 limit switch>"
  Supervisor/1(jogspeed_y_reset) -> Dct2lowpass yJogSpeed/1
  Dct2lowpass yJogSpeed/1 -> Discrete-Time Integrator x2JogSpeed1/1  "jogspeed_y_reset"
  Bus Selector/1 -> Supervisor/1(limitswitch_y)  "<DI carriage limit switch>"
  Discrete-Time Integrator x1JogSpeed/1 -> current_x4/2, current_x3/2
  Discrete-Time Integrator x2JogSpeed/1 -> current_x3/1, current_x4/1
  current_x4/1 -> Gain x2/1
  current_x3/1 -> Gain x3/1
  Gain x3/1 -> phiReset/1  "jogdistance_phi_reset"
  penholder_active/1 -> Supervisor/4(penholder_active)
  Supervisor/5(change_color) -> change_color/1
  Discrete-Time Integrator x2JogSpeed1/1 -> yReset/1  "jogdistance_y_reset"

== system Arizona_base_GOAT_TjeerdRC/Homing/Memory block for homing during trials/Memory_phi ==
  homeTrigger : Inport
  phiHome : Inport  Port=2
  Delay : Delay  DelayLength=1
  Delay1 : Delay  DelayLength=1
  Sum : Sum  Inputs=|++
  Switch : Switch  Criteria=u2 > Threshold  SaturateOnIntegerOverflow=off  InputSameDT=off
  Switch1 : Switch  Criteria=u2 > Threshold  SaturateOnIntegerOverflow=off  InputSameDT=off
  1 : Outport
  wires:
  Switch/1 -> Delay1/1  "Memory_loop_phi"
  phiHome/1 -> Sum/1
  Sum/1 -> Switch1/1  "main"
  Delay1/1 -> Switch/1, Switch1/3, Sum/2
  homeTrigger/1 -> Switch/2, Delay/1
  Delay/1 -> Switch1/2
  Switch1/1 -> Switch/3, 1/1

== system Arizona_base_GOAT_TjeerdRC/Homing/Memory block for homing during trials/Memory_x ==
  homeTrigger : Inport
  xHome : Inport  Port=2
  Delay : Delay  DelayLength=1
  Delay1 : Delay  DelayLength=1
  Sum : Sum  Inputs=|++
  Switch : Switch  Criteria=u2 > Threshold  SaturateOnIntegerOverflow=off  InputSameDT=off
  Switch1 : Switch  Criteria=u2 > Threshold  SaturateOnIntegerOverflow=off  InputSameDT=off
  1 : Outport
  wires:
  Switch/1 -> Delay1/1  "Memory_loop_x"
  xHome/1 -> Sum/1
  Sum/1 -> Switch1/1
  Delay1/1 -> Switch/1, Switch1/3, Sum/2
  homeTrigger/1 -> Switch/2, Delay/1
  Delay/1 -> Switch1/2
  Switch1/1 -> Switch/3, 1/1

== system Arizona_base_GOAT_TjeerdRC/Homing/Memory block for homing during trials/Memory_y ==
  homeTrigger : Inport
  yHome : Inport  Port=2
  Delay : Delay  DelayLength=1
  Delay1 : Delay  DelayLength=1
  Sum : Sum  Inputs=|++
  Switch : Switch  Criteria=u2 > Threshold  SaturateOnIntegerOverflow=off  InputSameDT=off
  Switch1 : Switch  Criteria=u2 > Threshold  SaturateOnIntegerOverflow=off  InputSameDT=off
  Out1 : Outport
  wires:
  Switch/1 -> Delay1/1  "Memory_loop_y"
  yHome/1 -> Sum/1
  Sum/1 -> Switch1/1
  Delay1/1 -> Switch/1, Switch1/3, Sum/2
  homeTrigger/1 -> Switch/2, Delay/1
  Delay/1 -> Switch1/2
  Switch1/1 -> Switch/3, Out1/1

== system Arizona_base_GOAT_TjeerdRC/Homing old/Enabled subsystem/Initialization ==
  Enable : EnablePort  StatesWhenEnabling=reset
  Compare To Constant NInit : simulink/Logic and Bit Operations/Compare To Constant  relop=>=  const=N_Init  OutDataTypeStr=boolean
  Counter Free-Running : simulink/Sources/Counter Free-Running  NumBits=32  tsamp=-1
  Data Type Conversion counter : DataTypeConversion  SaturateOnIntegerOverflow=off  RndMeth=Floor
  Data Type Conversion end trial : DataTypeConversion  SaturateOnIntegerOverflow=off  RndMeth=Floor
  Direct Lookup Table phiFF : LookupNDDirect  NumberOfTableDimensions=1  TableIsInput=on  Table=[4 5 ;16 19 ]
  Direct Lookup Table xFF : LookupNDDirect  NumberOfTableDimensions=1  TableIsInput=on  Table=[4 5 ;16 19 ]
  Direct Lookup Table yFF : LookupNDDirect  NumberOfTableDimensions=1  TableIsInput=on  Table=[4 5 ;16 19 ]
  set_phi_homing : Constant  Value=phi_Init
  set_x_homing : Constant  Value=x_Init
  set_y_homing : Constant  Value=y_Init
  yInit : Outport
  xInit : Outport  Port=2
  phiInit : Outport  Port=3
  initializationDone : Outport  Port=4
  wires:
  Data Type Conversion end trial/1 -> initializationDone/1  "h2"
  Compare To Constant NInit/1 -> Data Type Conversion end trial/1  "home_fin_check"
  Data Type Conversion counter/1 -> Direct Lookup Table xFF/1, Direct Lookup Table phiFF/1, Compare To Constant NInit/1, Direct Lookup Table yFF/1  "home_time"
  Counter Free-Running/1 -> Data Type Conversion counter/1
  set_phi_homing/1 -> Direct Lookup Table phiFF/2
  Direct Lookup Table xFF/1 -> xInit/1
  Direct Lookup Table yFF/1 -> yInit/1
  Direct Lookup Table phiFF/1 -> phiInit/1
  set_x_homing/1 -> Direct Lookup Table xFF/2
  set_y_homing/1 -> Direct Lookup Table yFF/2

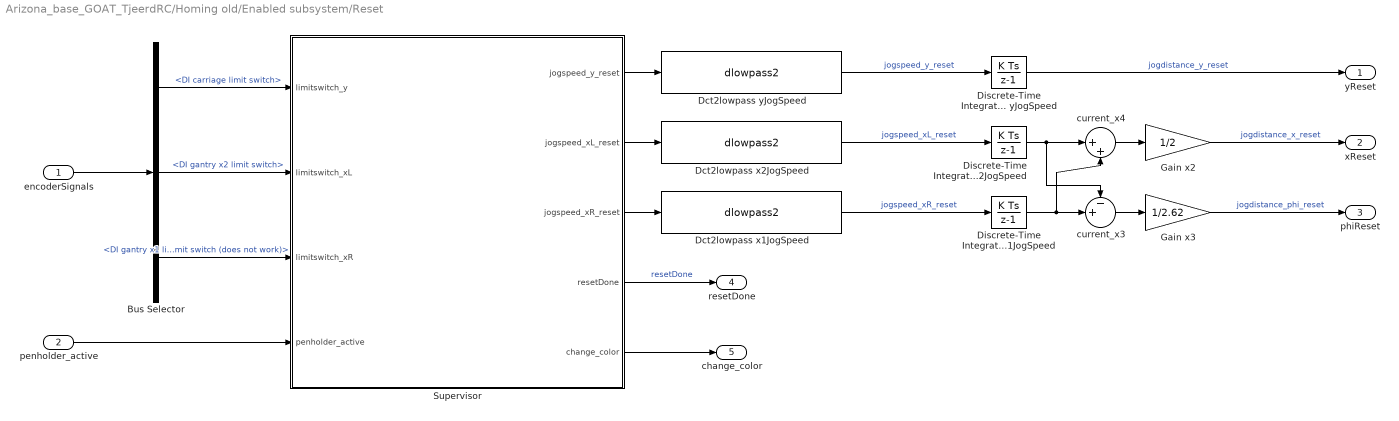
== system Arizona_base_GOAT_TjeerdRC/Homing old/Enabled subsystem/Reset ==
  encoderSignals : Inport
  penholder_active : Inport  Port=2
  Bus Selector : BusSelector  OutputSignals=DI limit switches.DI carriage limit switch,DI limit switches.DI gantry x2 limit switch,DI limit switches.DI gantry x1 limit switch (does not work)
  Dct2lowpass x1JogSpeed : S-Function  FunctionName=dlowpass2  Parameters=f_den, b_den, 0.001  SFunctionDeploymentMode=off  EnableBusSupport=off  mask(dctools){f_den=20, b_den=2}
      mask prompts: f_den "Pole [Hz]"; b_den "Damping pole [-]"
      mask help: This block implements a discrete time 2nd order lowpass filter.
      mask Display: disp('DCT 2nd order lowpass')
  Dct2lowpass x2JogSpeed : S-Function  FunctionName=dlowpass2  Parameters=f_den, b_den, 0.001  SFunctionDeploymentMode=off  EnableBusSupport=off  mask(dctools){f_den=20, b_den=2}
      mask prompts: f_den "Pole [Hz]"; b_den "Damping pole [-]"
      mask help: This block implements a discrete time 2nd order lowpass filter.
      mask Display: disp('DCT 2nd order lowpass')
  Dct2lowpass yJogSpeed : S-Function  FunctionName=dlowpass2  Parameters=f_den, b_den, 0.001  SFunctionDeploymentMode=off  EnableBusSupport=off  mask(dctools){f_den=10, b_den=1}
      mask prompts: f_den "Pole [Hz]"; b_den "Damping pole [-]"
      mask help: This block implements a discrete time 2nd order lowpass filter.
      mask Display: disp('DCT 2nd order lowpass')
  Discrete-Time Integrator x1JogSpeed : DiscreteIntegrator  SampleTime=-1  ICPrevOutput=DiscIntNeverNeededParam  ICPrevScaledInput=DiscIntNeverNeededParam
  Discrete-Time Integrator x2JogSpeed : DiscreteIntegrator  SampleTime=-1  ICPrevOutput=DiscIntNeverNeededParam  ICPrevScaledInput=DiscIntNeverNeededParam
  Discrete-Time Integrator yJogSpeed : DiscreteIntegrator  SampleTime=-1  ICPrevOutput=DiscIntNeverNeededParam  ICPrevScaledInput=DiscIntNeverNeededParam
  Gain x2 : Gain  Gain=1/2  OutDataTypeStr=double
  Gain x3 : Gain  Gain=1/2.62  OutDataTypeStr=double
  Supervisor : Stateflow chart  TreatAsAtomicUnit=on
  current_x3 : Sum  Inputs=-+|
  current_x4 : Sum  Inputs=|++
  yReset : Outport
  xReset : Outport  Port=2
  phiReset : Outport  Port=3
  resetDone : Outport  Port=4
  change_color : Outport  Port=5
  wires:
  Bus Selector/3 -> Supervisor/3(limitswitch_xR)  "<DI gantry x1 limit switch (does not work)>"
  Discrete-Time Integrator yJogSpeed/1 -> yReset/1  "jogdistance_y_reset"
  Gain x2/1 -> xReset/1  "jogdistance_x_reset"
  encoderSignals/1 -> Bus Selector/1
  Supervisor/4(resetDone) -> resetDone/1  "resetDone"
  Supervisor/2(jogspeed_xL_reset) -> Dct2lowpass x2JogSpeed/1
  Supervisor/3(jogspeed_xR_reset) -> Dct2lowpass x1JogSpeed/1
  Dct2lowpass x2JogSpeed/1 -> Discrete-Time Integrator x2JogSpeed/1  "jogspeed_xL_reset"
  Dct2lowpass x1JogSpeed/1 -> Discrete-Time Integrator x1JogSpeed/1  "jogspeed_xR_reset"
  Bus Selector/2 -> Supervisor/2(limitswitch_xL)  "<DI gantry x2 limit switch>"
  Supervisor/1(jogspeed_y_reset) -> Dct2lowpass yJogSpeed/1
  Dct2lowpass yJogSpeed/1 -> Discrete-Time Integrator yJogSpeed/1  "jogspeed_y_reset"
  Bus Selector/1 -> Supervisor/1(limitswitch_y)  "<DI carriage limit switch>"
  Discrete-Time Integrator x1JogSpeed/1 -> current_x4/2, current_x3/2
  Discrete-Time Integrator x2JogSpeed/1 -> current_x3/1, current_x4/1
  current_x4/1 -> Gain x2/1
  current_x3/1 -> Gain x3/1
  Gain x3/1 -> phiReset/1  "jogdistance_phi_reset"
  penholder_active/1 -> Supervisor/4(penholder_active)
  Supervisor/5(change_color) -> change_color/1

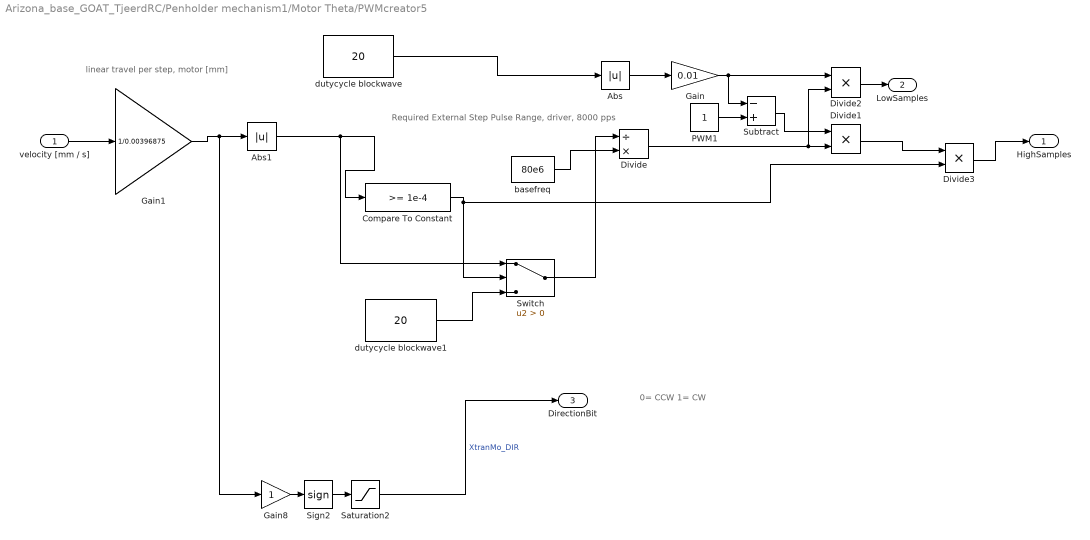
== system Arizona_base_GOAT_TjeerdRC/Penholder mechanism1/Motor Theta/PWMcreator5 ==
  note: Required External Step Pulse Range, driver, 8000 pps
  note: linear travel per step, motor [mm]
  note: 0= CCW
      | 1= CW
  velocity [mm / s] : Inport
  Abs : Abs  SaturateOnIntegerOverflow=off
  Abs1 : Abs  SaturateOnIntegerOverflow=off
  Compare To Constant : simulink/Logic and Bit Operations/Compare To Constant  relop=>=  const=1e-4  OutDataTypeStr=boolean
  Divide : Product  Inputs=/*
  Divide1 : Product  Inputs=**
  Divide2 : Product  Inputs=**
  Divide3 : Product  Inputs=**
  Gain : Gain  Gain=0.01
  Gain1 : Gain  Gain=1/0.00396875
  Gain8 : Gain
  PWM1 : Constant
  Saturation2 : Saturate  UpperLimit=1  LowerLimit=0
  Sign2 : Signum
  Subtract : Sum  Inputs=-+
  Switch : Switch  Criteria=u2 > Threshold  SaturateOnIntegerOverflow=off  InputSameDT=off
  basefreq : Constant  Value=80e6
  dutycycle blockwave : Constant  Value=20
  dutycycle blockwave1 : Constant  Value=20
  HighSamples : Outport
  LowSamples : Outport  Port=2
  DirectionBit : Outport  Port=3
  wires:
  Abs/1 -> Gain/1
  Sign2/1 -> Saturation2/1
  Gain8/1 -> Sign2/1
  Divide1/1 -> Divide3/1
  velocity [mm / s]/1 -> Gain1/1
  Divide2/1 -> LowSamples/1
  dutycycle blockwave/1 -> Abs/1
  PWM1/1 -> Subtract/2
  Subtract/1 -> Divide1/1
  Divide/1 -> Divide1/2, Divide2/2
  Gain/1 -> Subtract/1, Divide2/1
  basefreq/1 -> Divide/2
  Abs1/1 -> Compare To Constant/1, Switch/1
  Gain1/1 -> Gain8/1, Abs1/1
  Compare To Constant/1 -> Divide3/2, Switch/2
  Switch/1 -> Divide/1
  dutycycle blockwave1/1 -> Switch/3
  Divide3/1 -> HighSamples/1
  Saturation2/1 -> DirectionBit/1  "XtranMo_DIR"

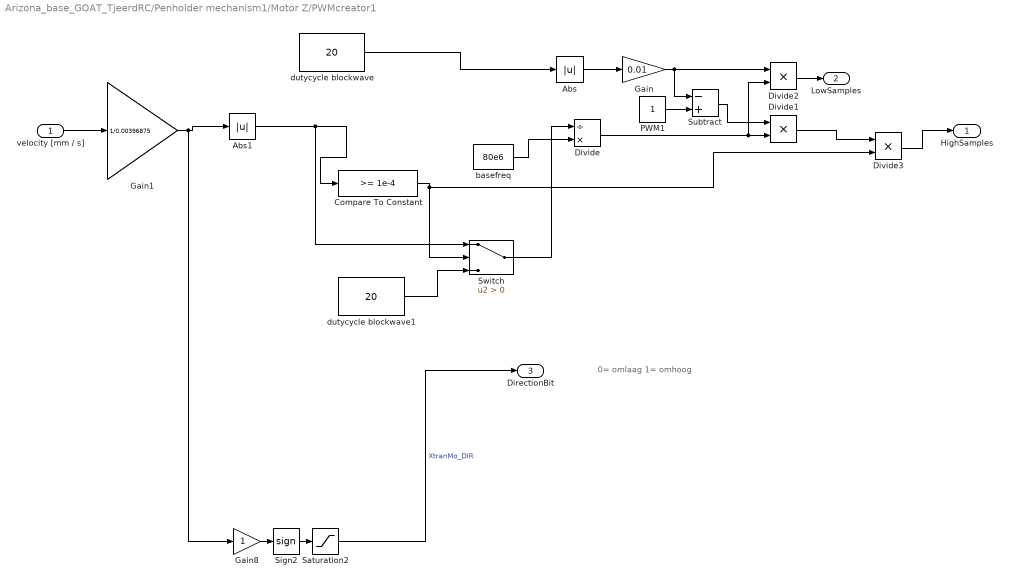
== system Arizona_base_GOAT_TjeerdRC/Penholder mechanism1/Motor Z/PWMcreator1 ==
  note: 0= omlaag
      | 1= omhoog
  velocity [mm / s] : Inport
  Abs : Abs  SaturateOnIntegerOverflow=off
  Abs1 : Abs  SaturateOnIntegerOverflow=off
  Compare To Constant : simulink/Logic and Bit Operations/Compare To Constant  relop=>=  const=1e-4  OutDataTypeStr=boolean
  Divide : Product  Inputs=/*
  Divide1 : Product  Inputs=**
  Divide2 : Product  Inputs=**
  Divide3 : Product  Inputs=**
  Gain : Gain  Gain=0.01
  Gain1 : Gain  Gain=1/0.00396875
  Gain8 : Gain
  PWM1 : Constant
  Saturation2 : Saturate  UpperLimit=1  LowerLimit=0
  Sign2 : Signum
  Subtract : Sum  Inputs=-+
  Switch : Switch  Criteria=u2 > Threshold  SaturateOnIntegerOverflow=off  InputSameDT=off
  basefreq : Constant  Value=80e6
  dutycycle blockwave : Constant  Value=20
  dutycycle blockwave1 : Constant  Value=20
  HighSamples : Outport
  LowSamples : Outport  Port=2
  DirectionBit : Outport  Port=3
  wires:
  Divide3/1 -> HighSamples/1
  dutycycle blockwave1/1 -> Switch/3
  Switch/1 -> Divide/1
  Compare To Constant/1 -> Switch/2, Divide3/2
  Gain1/1 -> Gain8/1, Abs1/1
  Abs1/1 -> Switch/1, Compare To Constant/1
  basefreq/1 -> Divide/2
  Gain/1 -> Divide2/1, Subtract/1
  Divide/1 -> Divide2/2, Divide1/2
  Subtract/1 -> Divide1/1
  PWM1/1 -> Subtract/2
  dutycycle blockwave/1 -> Abs/1
  Divide2/1 -> LowSamples/1
  velocity [mm / s]/1 -> Gain1/1
  Divide1/1 -> Divide3/1
  Gain8/1 -> Sign2/1
  Sign2/1 -> Saturation2/1
  Abs/1 -> Gain/1
  Saturation2/1 -> DirectionBit/1  "XtranMo_DIR"

== stateflow chart Arizona_base_GOAT_TjeerdRC/Trial control with Penholder enabling ==
  state TRIAL_FINISHED
    en:
    trialTrigger=0;
    change_color=0;
  state PEN_CHANGING
  state idle
    en:
    trialTrigger = 0;
  state initialization
  state PEN_READY
    en:
    change_color=0;
  state trial
    en:
    trialTrigger = 1;
    timeIndex = 0;
    trialIndex++;
    du:
    timeIndex++;
  idle -> PEN_CHANGING [order 1] : [startPenholder==1 && PenColor == 1]
      | {change_color=6}
  TRIAL_FINISHED -> PEN_CHANGING : [after(0.1,sec)]
      | {change_color=PenColor}
  idle -> PEN_CHANGING [order 2] : [startPenholder==1 && PenColor ~= 1]
      | {change_color = PenColor}
  PEN_CHANGING -> PEN_READY : [after(0.1,sec) && penholder_active==0]
  trial -> TRIAL_FINISHED : %Transition if trial is ended.
      | [TrialDone]
  initialization -> idle : %Transition if initialization is completed.
      | [homingDone]
  (default) -> initialization
  PEN_READY -> idle [order 2] : [startPenholder==0]{change_color=5}
  PEN_READY -> trial [order 1] : %Start ILC trial
      | [startTrial]
  data: homingDone input double; startTrial input double; startPenholder input; trialTrigger output double =0; timeIndex local double =0; Nref parameter double; trialIndex output double =0; TrialDone input; change_color output double; penholder_active input; PenColor input

== stateflow chart Arizona_base_GOAT_TjeerdRC/Homing old/Enabled subsystem/Reset/Supervisor ==
  state MOVE_PEN_UP
    entry:
    change_color=5;
  state PEN_READY
    entry:
    change_color=0;
  state MoveToLimitSwitches
    state reset_gantryLeft [parallel]
      settings: executionOrder=1
      state increase_jogspeed
        during:
        jogspeed_xL_reset = max(-0.10,jogspeed_xL_reset - 0.10*Ts/1);
      state stop
        entry:
        jogspeed_xL_reset = 0;
      (default) -> MoveToLimitSwitches.reset_gantryLeft.increase_jogspeed
      MoveToLimitSwitches.reset_gantryLeft.increase_jogspeed -> MoveToLimitSwitches.reset_gantryLeft.stop : [limitswitch_xL]
    state reset_gantryright [parallel]
      settings: executionOrder=2
      state increase_jogspeed
        during:
        jogspeed_xR_reset = max(-0.10,jogspeed_xR_reset - 0.10*Ts/1);
      state stop
        entry:
        jogspeed_xR_reset = 0;
      (default) -> MoveToLimitSwitches.reset_gantryright.increase_jogspeed
      MoveToLimitSwitches.reset_gantryright.increase_jogspeed -> MoveToLimitSwitches.reset_gantryright.stop : [limitswitch_xL]
    state reset_carriage [parallel]
      settings: executionOrder=3
      state increase_jogspeed
        during:
        jogspeed_y_reset = max(-0.25,jogspeed_y_reset - 0.25*Ts/1);
      state stop
        entry:
        jogspeed_y_reset = 0;
      (default) -> MoveToLimitSwitches.reset_carriage.increase_jogspeed
      MoveToLimitSwitches.reset_carriage.increase_jogspeed -> MoveToLimitSwitches.reset_carriage.stop : [limitswitch_y]
  state enablePointToRefs
    entry:
    resetDone = true;
  (default) -> MOVE_PEN_UP
  MOVE_PEN_UP -> PEN_READY : [after(1,sec) && penholder_active==0]
  PEN_READY -> MoveToLimitSwitches
  MoveToLimitSwitches -> enablePointToRefs : [(jogspeed_xL_reset==0) && (jogspeed_xR_reset==0) && (jogspeed_y_reset==0)]
  data: jogspeed_y_reset output double =-0.25*Ts/1; jogspeed_xL_reset output double =-0.10*Ts/1; limitswitch_y input double; limitswitch_xL input double; limitswitch_xR input double; jogspeed_xR_reset output double =-0.10*Ts/1; resetDone output double =0; Ts local double =Ts; penholder_active input; change_color output double
